simulink model "GMCLIB_ElimDcBusRip_BAM_F32"  (Simulink 8.3)
settings: Solver=ode45  StartTime=0.0  StopTime=10.0  RelTol=1e-3
undefined symbols (not defined in the file): f32ModIndex
settings Model: Creator=B17364  LastModifiedBy=B17364
settings DataIOCC: SignalLoggingSaveFormat=Dataset
settings DebuggingCC: UnderspecifiedInitializationDetection=Simplified  StateNameClashWarn=none
settings GRTTargetCC: CombineOutputUpdateFcns=on  GRTInterface=off

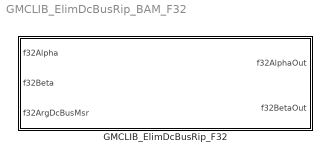
== system GMCLIB_ElimDcBusRip_BAM_F32 ==
  GMCLIB_ElimDcBusRip_F32 : Subsystem  mask(GMCLIB_ElimDcBusRip_F32){f32ModIndex=f32ModIndex}
      mask help: Bit accurate model of DC Bus voltage ripple elimination function.
      mask init:
      | pos = get_param(gcb, 'Position');width = pos(3) - pos(1); height = pos(4) - pos(2);tX=width/2;tY=height*0.9;
      mask Display: color('black');port_label('input',1,'f32Alpha');port_label('input',2,'f32Beta');port_label('input',3,'f32ArgDcBusMsr');port_label('output',1,'f32AlphaOut');port_label('output',2,'f32BetaOut');color('black');disp('GMCLIB_ElimDcBusRip_F32');color('blue');text(tX,tY, 'BAM', 'horizontalAlignment', 'center');

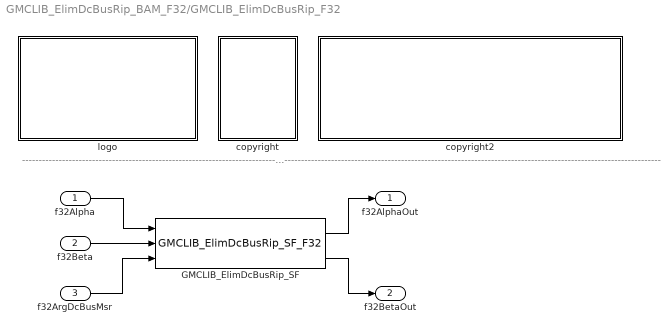
== system GMCLIB_ElimDcBusRip_BAM_F32/GMCLIB_ElimDcBusRip_F32 ==
  note: ---------------------------------------------------------------------------------------------------------------------------------------------------------------------------------------------------
  f32Alpha : Inport
  f32Beta : Inport  Port=2
  f32ArgDcBusMsr : Inport  Port=3
  GMCLIB_ElimDcBusRip_SF : S-Function  FunctionName=GMCLIB_ElimDcBusRip_SF_F32  Parameters=f32ModIndex  EnableBusSupport=off
  copyright : Subsystem
      mask Display: text(10,90,'FILE:');text(10,75,'DESRIPTION:');text(10,60,'COPYRIGHT:');text(10,45,'VERSION:');text(10,30,'DATE:')
  copyright2 : Subsystem
      mask Display: text(10,90,'GMCLIB_ElimDcBusRip_BAM_F32.mdl');text(10,75,'DC Bus voltage ripple elimination function.');text(10,60,'Freescale');text(10,45,'0.1');text(10,30,'12-Jun-2015');
  logo : Subsystem
      mask Display: image(imread('logo.jpg'))
  f32AlphaOut : Outport
  f32BetaOut : Outport  Port=2
  wires:
  f32Alpha/1 -> GMCLIB_ElimDcBusRip_SF/1
  f32Beta/1 -> GMCLIB_ElimDcBusRip_SF/2
  f32ArgDcBusMsr/1 -> GMCLIB_ElimDcBusRip_SF/3
  GMCLIB_ElimDcBusRip_SF/1 -> f32AlphaOut/1
  GMCLIB_ElimDcBusRip_SF/2 -> f32BetaOut/1

== system GMCLIB_ElimDcBusRip_BAM_F32/GMCLIB_ElimDcBusRip_F32/copyright ==

== system GMCLIB_ElimDcBusRip_BAM_F32/GMCLIB_ElimDcBusRip_F32/copyright2 ==

== system GMCLIB_ElimDcBusRip_BAM_F32/GMCLIB_ElimDcBusRip_F32/logo ==
